simulink model "lab4_1_2"  (R2022a)
settings: Solver=VariableStepAuto  StartTime=0.0  StopTime=Tmdl  FixedStep=To/100  MaxStep=To/100  RelTol=1e-3
undefined symbols (not defined in the file or in its folder): an, dsc, T, To
settings Model: Creator=Professional  LastModifiedBy=osini

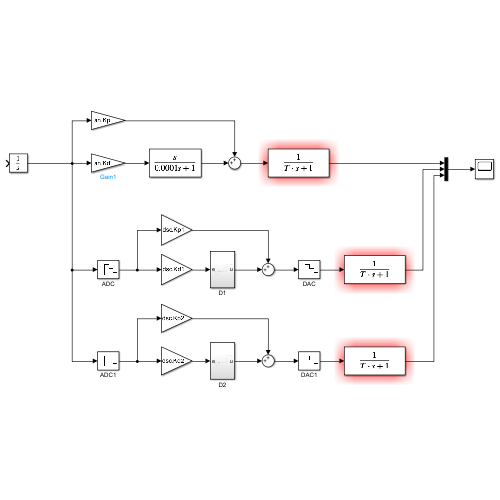
[thumbnail: Simulink's stored preview of the top-level diagram]
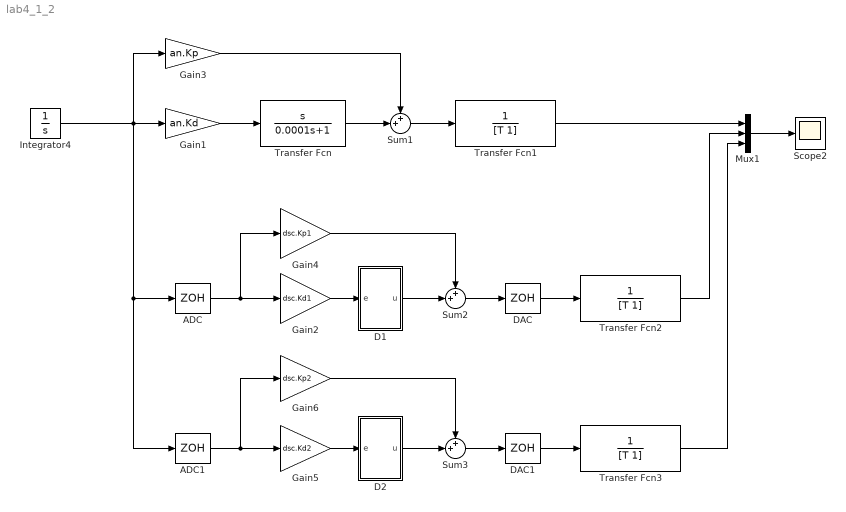
== system lab4_1_2 ==
  ADC : ZeroOrderHold  SampleTime=To
  ADC1 : ZeroOrderHold  SampleTime=To
  D1 : Subsystem
  D2 : Subsystem
  DAC : ZeroOrderHold  SampleTime=To
  DAC1 : ZeroOrderHold  SampleTime=To
  Gain1 : Gain  Gain=an.Kd
  Gain2 : Gain  Gain=dsc.Kd1
  Gain3 : Gain  Gain=an.Kp
  Gain4 : Gain  Gain=dsc.Kp1
  Gain5 : Gain  Gain=dsc.Kd2
  Gain6 : Gain  Gain=dsc.Kp2
  Integrator4 : Integrator  InitialCondition=1
  Mux1 : Mux  Inputs=3
  Scope2 : Scope
  Sum1 : Sum  Inputs=++|
  Sum2 : Sum  Inputs=++|
  Sum3 : Sum  Inputs=++|
  Transfer Fcn : TransferFcn  Numerator=[1 0]  Denominator=[0.0001 1]
  Transfer Fcn1 : TransferFcn  Denominator=[T 1]
  Transfer Fcn2 : TransferFcn  Denominator=[T 1]
  Transfer Fcn3 : TransferFcn  Denominator=[T 1]
  wires:
  Mux1/1 -> Scope2/1
  Gain1/1 -> Transfer Fcn/1
  Transfer Fcn/1 -> Sum1/2
  Gain3/1 -> Sum1/1
  Sum1/1 -> Transfer Fcn1/1
  Transfer Fcn1/1 -> Mux1/1
  Sum2/1 -> DAC/1
  D1/1(u) -> Sum2/2
  Gain4/1 -> Sum2/1
  ADC/1 -> Gain4/1, Gain2/1
  Gain2/1 -> D1/1(e)
  DAC/1 -> Transfer Fcn2/1
  Transfer Fcn2/1 -> Mux1/2
  ADC1/1 -> Gain6/1, Gain5/1
  Transfer Fcn3/1 -> Mux1/3
  Gain5/1 -> D2/1(e)
  Integrator4/1 -> ADC1/1, ADC/1, Gain3/1, Gain1/1
  DAC1/1 -> Transfer Fcn3/1
  Gain6/1 -> Sum3/1
  D2/1(u) -> Sum3/2
  Sum3/1 -> DAC1/1

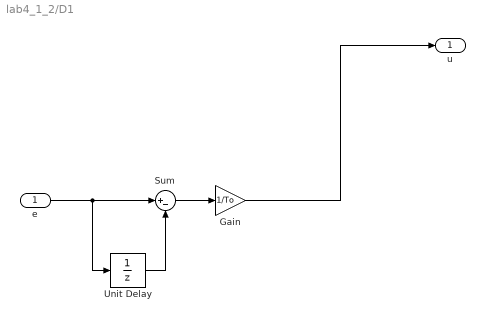
== system lab4_1_2/D1 ==
  e : Inport
  Gain : Gain  Gain=1/To
  Sum : Sum  Inputs=|+-
  Unit Delay : UnitDelay  SampleTime=-1  HasFrameUpgradeWarning=on
  u : Outport
  wires:
  e/1 -> Unit Delay/1, Sum/1
  Unit Delay/1 -> Sum/2
  Gain/1 -> u/1
  Sum/1 -> Gain/1

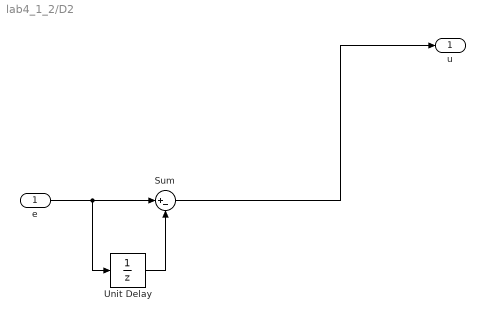
== system lab4_1_2/D2 ==
  e : Inport
  Sum : Sum  Inputs=|+-
  Unit Delay : UnitDelay  SampleTime=-1  HasFrameUpgradeWarning=on
  u : Outport
  wires:
  e/1 -> Unit Delay/1, Sum/1
  Unit Delay/1 -> Sum/2
  Sum/1 -> u/1
